simulink model "untitled"  (R2021a)
settings: Solver=VariableStepAuto  StartTime=0.0  StopTime=100  RelTol=1e-3
settings Model: Creator=OMEN  LastModifiedBy=OMEN

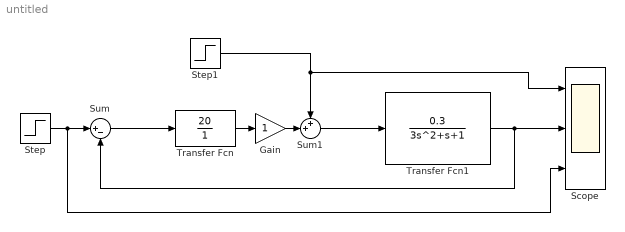
== system untitled ==
  Gain : Gain
  Scope : Scope  NumInputPorts=3
  Step : Step  SampleTime=0
  Step1 : Step  Before=1  SampleTime=0
  Sum : Sum  Inputs=|+-
  Sum1 : Sum  Inputs=++|
  Transfer Fcn : TransferFcn  Numerator=[20]  Denominator=[1]
  Transfer Fcn1 : TransferFcn  Numerator=[0.3]  Denominator=[3 1 1]
  wires:
  Step/1 -> Scope/3, Sum/1
  Sum/1 -> Transfer Fcn/1
  Step1/1 -> Scope/1, Sum1/1
  Transfer Fcn1/1 -> Sum/2, Scope/2
  Sum1/1 -> Transfer Fcn1/1
  Transfer Fcn/1 -> Gain/1
  Gain/1 -> Sum1/2
